simulink model "HIL"  (R2019a)
settings: configuration reference "Configuration" (kept outside this file)
undefined symbols (not defined in the file): Ts
libraries: aerolibutil x2, vrlib x1
settings Model: Creator=zouji  LastModifiedBy=Bingo
settings ConfigSetRef: SourceName=Configuration  SourceLocation=Base Workspace

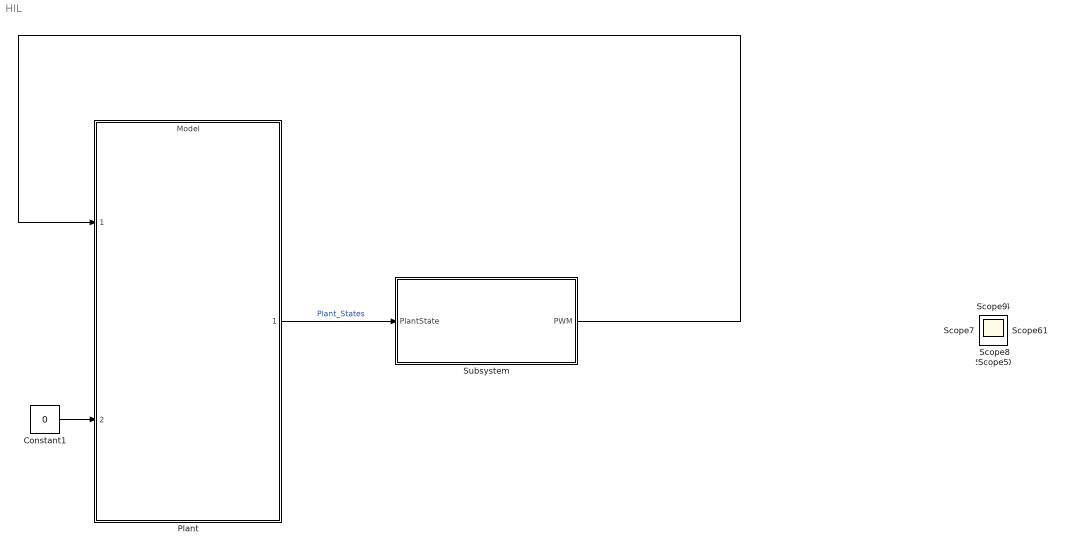
== system HIL ==
  Constant1 : Constant  Value=0  OutDataTypeStr=Inherit: Inherit via back propagation
  Plant : ModelReference  ModelNameDialog=Model.slx  SimulationMode=Normal  ModelReferenceVersion=1.125
  Subsystem : Subsystem
  Scope{,1..11} (12 alike) : Scope
  wires:
  Constant1/1 -> Plant/2
  Subsystem/1(PWM) -> Plant/1
  Plant/1 -> Subsystem/1(PlantState)  "Plant_States"

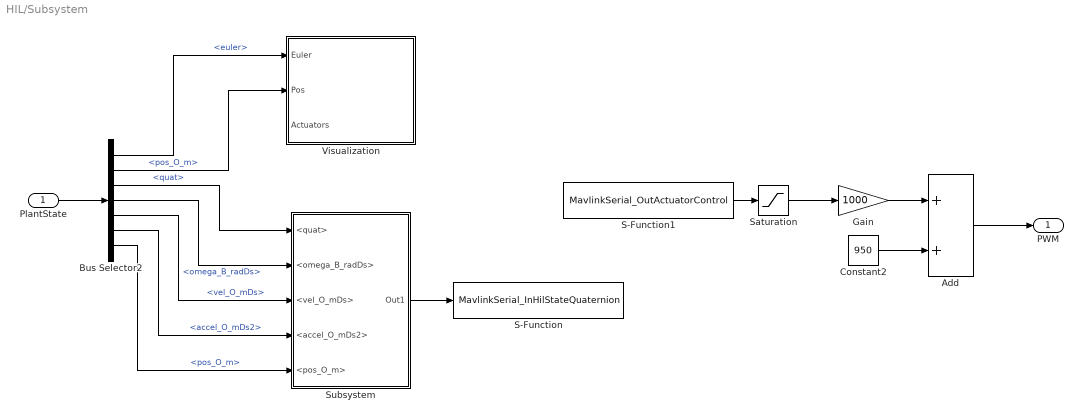
== system HIL/Subsystem ==
  PlantState : Inport
  Add : Sum
  Bus Selector2 : BusSelector  OutputSignals=euler,pos_O_m,quat,omega_B_radDs,vel_O_mDs,accel_O_mDs2,pos_O_m
  Constant2 : Constant  Value=950  OutDataTypeStr=uint16
  Gain : Gain  Gain=1000  OutDataTypeStr=uint16
  S-Function : S-Function  FunctionName=MavlinkSerial_InHilStateQuaternion  SFunctionDeploymentMode=off  EnableBusSupport=off
  S-Function1 : S-Function  FunctionName=MavlinkSerial_OutActuatorControl  SFunctionDeploymentMode=off  EnableBusSupport=off
  Saturation : Saturate  UpperLimit=1  LowerLimit=0
  Subsystem : Subsystem
  Visualization : Subsystem
  PWM : Outport
  wires:
  Add/1 -> PWM/1
  Saturation/1 -> Gain/1
  Constant2/1 -> Add/2
  Gain/1 -> Add/1
  PlantState/1 -> Bus Selector2/1
  S-Function1/1 -> Saturation/1
  Bus Selector2/1 -> Visualization/1(Euler)  "<euler>"
  Bus Selector2/2 -> Visualization/2(Pos)  "<pos_O_m>"
  Bus Selector2/3 -> Subsystem/1(<quat>)  "<quat>"
  Bus Selector2/4 -> Subsystem/2(<omega_B_radDs>)  "<omega_B_radDs>"
  Bus Selector2/5 -> Subsystem/3(<vel_O_mDs>)  "<vel_O_mDs>"
  Bus Selector2/6 -> Subsystem/4(<accel_O_mDs2>)  "<accel_O_mDs2>"
  Bus Selector2/7 -> Subsystem/5(<pos_O_m>)  "<pos_O_m>"
  Subsystem/1(Out1) -> S-Function/1

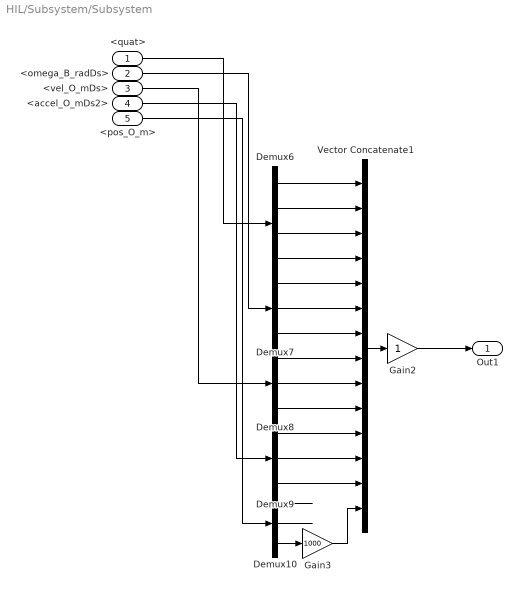
== system HIL/Subsystem/Subsystem ==
  <quat> : Inport
  <omega_B_radDs> : Inport  Port=2
  <vel_O_mDs> : Inport  Port=3
  <accel_O_mDs2> : Inport  Port=4
  <pos_O_m> : Inport  Port=5
  Demux{7..10} (4 alike) : Demux  Outputs=3
  Demux6 : Demux
  Gain2 : Gain  OutDataTypeStr=double
  Gain3 : Gain  Gain=1000
  Vector Concatenate1 : Concatenate  NumInputs=14
  Out1 : Outport
  wires:
  Demux9/2 -> Vector Concatenate1/12
  Gain3/1 -> Vector Concatenate1/14
  Demux6/4 -> Vector Concatenate1/4
  Demux9/1 -> Vector Concatenate1/11
  Gain2/1 -> Out1/1
  Demux8/1 -> Vector Concatenate1/8
  Demux10/3 -> Gain3/1
  Demux9/3 -> Vector Concatenate1/13
  Demux6/1 -> Vector Concatenate1/1
  Demux8/3 -> Vector Concatenate1/10
  Demux7/3 -> Vector Concatenate1/7
  Demux7/1 -> Vector Concatenate1/5
  Vector Concatenate1/1 -> Gain2/1
  Demux7/2 -> Vector Concatenate1/6
  Demux6/3 -> Vector Concatenate1/3
  Demux8/2 -> Vector Concatenate1/9
  Demux10/1 -> ?
  Demux6/2 -> Vector Concatenate1/2
  Demux10/2 -> ?
  <pos_O_m>/1 -> Demux10/1
  <quat>/1 -> Demux6/1
  <vel_O_mDs>/1 -> Demux8/1
  <omega_B_radDs>/1 -> Demux7/1
  <accel_O_mDs2>/1 -> Demux9/1

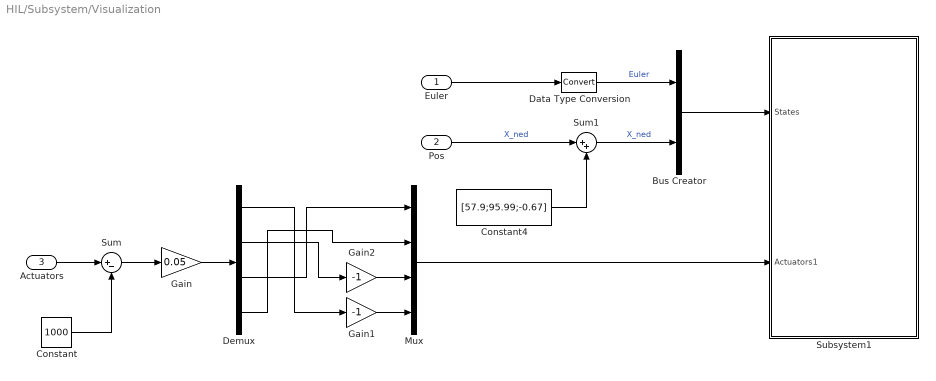
== system HIL/Subsystem/Visualization ==
  Euler : Inport
  Pos : Inport  Port=2
  Actuators : Inport  Port=3
  Bus Creator : BusCreator  Inputs=2
  Constant : Constant  Value=1000  OutDataTypeStr=uint16
  Constant4 : Constant  Value=[57.9;95.99;-0.67]  OutDataTypeStr=Inherit: Inherit via back propagation
  Data Type Conversion : DataTypeConversion
  Demux : Demux
  Gain : Gain  Gain=0.05  OutDataTypeStr=Inherit: Same as input
  Gain1 : Gain  Gain=-1  OutDataTypeStr=Inherit: Same as input
  Gain2 : Gain  Gain=-1  OutDataTypeStr=Inherit: Same as input
  Mux : Mux
  Subsystem1 : Subsystem
  Sum : Sum  Inputs=|+-  OutDataTypeStr=single
  Sum1 : Sum  Inputs=|++
  wires:
  Bus Creator/1 -> Subsystem1/1(States)
  Euler/1 -> Data Type Conversion/1
  Sum1/1 -> Bus Creator/2  "X_ned"
  Actuators/1 -> Sum/1
  Constant/1 -> Sum/2
  Sum/1 -> Gain/1
  Gain/1 -> Demux/1
  Demux/1 -> Gain1/1
  Gain1/1 -> Mux/4
  Demux/2 -> Gain2/1
  Demux/3 -> Mux/1
  Demux/4 -> Mux/2
  Gain2/1 -> Mux/3
  Mux/1 -> Subsystem1/2(Actuators1)
  Constant4/1 -> Sum1/2
  Pos/1 -> Sum1/1  "X_ned"
  Data Type Conversion/1 -> Bus Creator/1  "Euler"

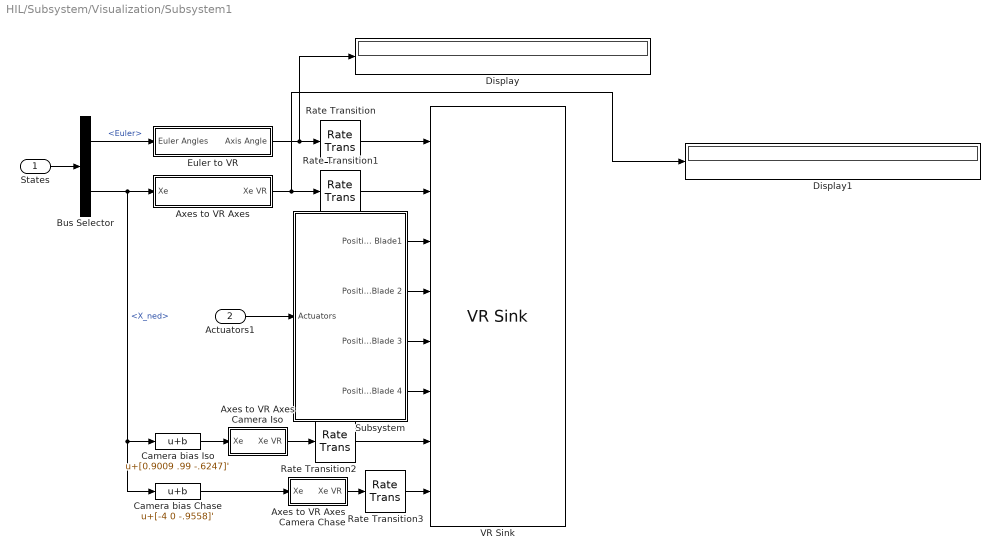
== system HIL/Subsystem/Visualization/Subsystem1 ==
  States : Inport
  Actuators1 : Inport  Port=2
  Axes to VR Axes : Subsystem
  Axes to VR Axes Camera Chase : Subsystem
  Axes to VR Axes Camera Iso : Subsystem
  Bus Selector : BusSelector  OutputSignals=Euler,X_ned
  Camera bias Chase : Bias  Bias=[-4 0 -.9558]'
  Camera bias Iso : Bias  Bias=[0.9009 .99 -.6247]'
  Display : Display
  Display1 : Display
  Euler to VR : Subsystem
  Rate Transition{,1..3} (4 alike) : RateTransition
  Subsystem : Subsystem
  VR Sink : vrlib/VR Sink  InstantiateOnLoad=on  SampleTime=12*Ts  ViewEnable=on  RemoteChange=off  RemoteView=off  FieldsWritten=QuadBody.rotation.4.1.1.double#QuadBody.translation.3.1.1.double#Blade1.rotation.4.1.1.double#Blade3.rotation.4.1.1.double#Blade2.rotation.4.1.1.double#Blade4.rotation.4.1.1.double#IsoNoRotation.position.3.1.1.double#OnQuadNoRotation.position.3.1.1.double  WorldFileName=asbQuadcopterWorld.wrl  AutoView=on  VideoDimensions=[]  AllowVariableSize=off  FigureProperties="{'Position', 'Name', 'Viewpoint', 'CameraBound', 'CameraDirection', 'CameraPosition', 'CameraUpVector', 'ZoomFactor', 'Antialiasing', 'Headlight', 'Lighting', 'NavPanel', 'Sound', 'StatusBar', 'Stereo3D', 'Stereo3DCameraOffset', 'Stereo3DHIT', 'ToolBar', 'Textures', 'Transparency', 'Triad', 'Wireframe', 'NavZones', 'NavMode', 'NavSpeed', 'CaptureFileFormat', 'CaptureFileName', 'Record2DCompressMethod', 'Record2DCompressQuality', 'Record2D', 'Record2DFileName', 'Record2DFPS'; [-1.9190000000000000e+03   1.7500000000000000e+02   1.9200000000000000e+03   9.2200000000000000e+02], '', 'Chase - No Rotation', 'on', [0.0000000000000000e+00   0.0000000000000000e+00  -1.0000000000000000e+00], [0.0000000000000000e+00   0.0000000000000000e+00   0.0000000000000000e+00], [0.0000000000000000e+00   1.0000000000000000e+00   0.0000000000000000e+00], [1.0000000000000000e+00], 'on', 'on', 'on', 'halfbar', 'on', 'on', 'off', [1.0000000149011612e-01], [0.0000000000000000e+00], 'on', 'on', 'on', 'none', 'off', 'off', 'fly', 'normal', 'tif', '%f_anim_%n.tif', 'auto', [7.5000000000000000e+01], 'off', '%f_anim_%n.avi', 'auto'}"
      settings: SourceProductBaseCode=VR
  wires:
  Rate Transition/1 -> VR Sink/1
  Subsystem/3(Position Blade 3) -> VR Sink/5
  States/1 -> Bus Selector/1
  Subsystem/4(Position Blade 4) -> VR Sink/6
  Bus Selector/1 -> Euler to VR/1(Euler Angles)  "<Euler>"
  Camera bias Iso/1 -> Axes to VR Axes Camera Iso/1(Xe)
  Axes to VR Axes/1(Xe VR) -> Display1/1, Rate Transition1/1
  Rate Transition1/1 -> VR Sink/2
  Axes to VR Axes Camera Iso/1(Xe VR) -> Rate Transition2/1
  Bus Selector/2 -> Camera bias Chase/1, Camera bias Iso/1, Axes to VR Axes/1(Xe)  "<X_ned>"
  Axes to VR Axes Camera Chase/1(Xe VR) -> Rate Transition3/1
  Subsystem/2(Position Blade 2) -> VR Sink/4
  Actuators1/1 -> Subsystem/1(Actuators)
  Subsystem/1(Position Blade1) -> VR Sink/3
  Euler to VR/1(Axis Angle) -> Display/1, Rate Transition/1
  Rate Transition3/1 -> VR Sink/8
  Rate Transition2/1 -> VR Sink/7
  Camera bias Chase/1 -> Axes to VR Axes Camera Chase/1(Xe)

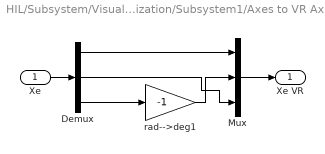
== system HIL/Subsystem/Visualization/Subsystem1/Axes to VR Axes ==
  Xe : Inport
  Demux : Demux  Outputs=3
  Mux : Mux  Inputs=3
  rad-->deg1 : Gain  Gain=-1  SaturateOnIntegerOverflow=on  OutDataTypeStr=Inherit: Same as input  ParamDataTypeStr=Inherit: Same as input
  Xe VR : Outport
  wires:
  Xe/1 -> Demux/1
  Demux/1 -> Mux/1
  Demux/3 -> rad-->deg1/1
  Mux/1 -> Xe VR/1
  rad-->deg1/1 -> Mux/2
  Demux/2 -> Mux/3

== system HIL/Subsystem/Visualization/Subsystem1/Axes to VR Axes Camera Chase ==
  Xe : Inport
  Demux : Demux  Outputs=3
  Mux : Mux  Inputs=3
  rad-->deg1 : Gain  Gain=-1  SaturateOnIntegerOverflow=on  OutDataTypeStr=Inherit: Same as input  ParamDataTypeStr=Inherit: Same as input
  Xe VR : Outport
  wires:
  Xe/1 -> Demux/1
  Demux/1 -> Mux/1
  Demux/3 -> rad-->deg1/1
  Mux/1 -> Xe VR/1
  rad-->deg1/1 -> Mux/2
  Demux/2 -> Mux/3

== system HIL/Subsystem/Visualization/Subsystem1/Axes to VR Axes Camera Iso ==
  Xe : Inport
  Demux : Demux  Outputs=3
  Mux : Mux  Inputs=3
  rad-->deg1 : Gain  Gain=-1  SaturateOnIntegerOverflow=on  OutDataTypeStr=Inherit: Same as input  ParamDataTypeStr=Inherit: Same as input
  Xe VR : Outport
  wires:
  Demux/2 -> Mux/3
  rad-->deg1/1 -> Mux/2
  Mux/1 -> Xe VR/1
  Demux/3 -> rad-->deg1/1
  Demux/1 -> Mux/1
  Xe/1 -> Demux/1

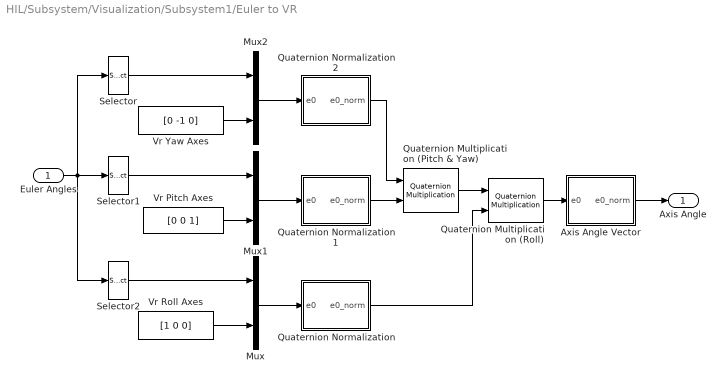
== system HIL/Subsystem/Visualization/Subsystem1/Euler to VR ==
  Euler Angles : Inport
  Axis Angle Vector : Subsystem
  Mux : Mux  Inputs=2
  Mux1 : Mux  Inputs=2
  Mux2 : Mux  Inputs=2
  Quaternion Multiplication (Pitch & Yaw) : aerolibutil/Quaternion Multiplication
  Quaternion Multiplication (Roll) : aerolibutil/Quaternion Multiplication
  Quaternion Normalization : Subsystem
  Quaternion Normalization1 : Subsystem
  Quaternion Normalization2 : Subsystem
  Selector : Selector  InputPortWidth=3  IndexOptions=Index vector (dialog)  Indices=[3]  OutputSizes=1
  Selector1 : Selector  InputPortWidth=3  IndexOptions=Index vector (dialog)  Indices=[2]  OutputSizes=1
  Selector2 : Selector  InputPortWidth=3  IndexOptions=Index vector (dialog)  Indices=[1]  OutputSizes=1
  Vr Pitch Axes : Constant  Value=[0 0 1]
  Vr Roll Axes : Constant  Value=[1 0 0]
  Vr Yaw Axes : Constant  Value=[0 -1 0]
  Axis Angle : Outport
  wires:
  Quaternion Multiplication (Roll)/1 -> Axis Angle Vector/1(e0)
  Axis Angle Vector/1(e0_norm) -> Axis Angle/1
  Quaternion Normalization/1(e0_norm) -> Quaternion Multiplication (Roll)/2
  Quaternion Normalization2/1(e0_norm) -> Quaternion Multiplication (Pitch & Yaw)/1
  Quaternion Normalization1/1(e0_norm) -> Quaternion Multiplication (Pitch & Yaw)/2
  Mux2/1 -> Quaternion Normalization2/1(e0)
  Mux1/1 -> Quaternion Normalization1/1(e0)
  Mux/1 -> Quaternion Normalization/1(e0)
  Selector/1 -> Mux2/1
  Vr Yaw Axes/1 -> Mux2/2
  Selector1/1 -> Mux1/1
  Vr Pitch Axes/1 -> Mux1/2
  Selector2/1 -> Mux/1
  Vr Roll Axes/1 -> Mux/2
  Euler Angles/1 -> Selector2/1, Selector1/1, Selector/1
  Quaternion Multiplication (Pitch & Yaw)/1 -> Quaternion Multiplication (Roll)/1

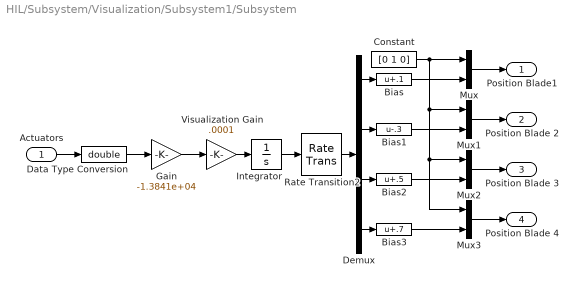
== system HIL/Subsystem/Visualization/Subsystem1/Subsystem ==
  Actuators : Inport
  Bias : Bias  Bias=.1
  Bias1 : Bias  Bias=-.3
  Bias2 : Bias  Bias=.5
  Bias3 : Bias  Bias=.7
  Constant : Constant  Value=[0 1 0]
  Data Type Conversion : DataTypeConversion  OutDataTypeStr=double
  Demux : Demux
  Gain : Gain  Gain=-1.3841e+04
  Integrator : Integrator  InitialCondition="[.1  .2 -.3 -.4]"  WrapState=on  WrappedStateUpperValue=2*pi  WrappedStateLowerValue=-2*pi
  Mux{,1..3} (4 alike) : Mux  Inputs=2
  Rate Transition2 : RateTransition
  Visualization Gain : Gain  Gain=.0001
  Position Blade1 : Outport
  Position Blade 2 : Outport  Port=2
  Position Blade 3 : Outport  Port=3
  Position Blade 4 : Outport  Port=4
  wires:
  Bias3/1 -> Mux3/2
  Mux3/1 -> Position Blade 4/1
  Bias1/1 -> Mux1/2
  Bias2/1 -> Mux2/2
  Demux/2 -> Bias1/1
  Visualization Gain/1 -> Integrator/1
  Constant/1 -> Mux3/1, Mux2/1, Mux1/1, Mux/1
  Mux1/1 -> Position Blade 2/1
  Mux2/1 -> Position Blade 3/1
  Data Type Conversion/1 -> Gain/1
  Integrator/1 -> Rate Transition2/1
  Mux/1 -> Position Blade1/1
  Gain/1 -> Visualization Gain/1
  Demux/3 -> Bias2/1
  Bias/1 -> Mux/2
  Actuators/1 -> Data Type Conversion/1
  Demux/4 -> Bias3/1
  Rate Transition2/1 -> Demux/1
  Demux/1 -> Bias/1

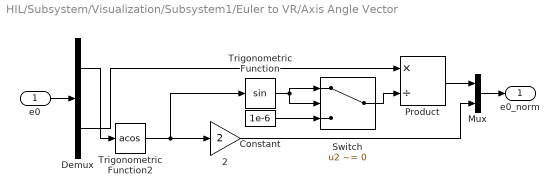
== system HIL/Subsystem/Visualization/Subsystem1/Euler to VR/Axis Angle Vector ==
  e0 : Inport
  2 : Gain  Gain=2  SaturateOnIntegerOverflow=on  OutDataTypeStr=Inherit: Same as input  ParamDataTypeStr=Inherit: Same as input
  Constant : Constant  Value=1e-6
  Demux : Demux  Outputs=[1 3 ]
  Mux : Mux  Inputs=2
  Product : Product  Inputs=*/  SaturateOnIntegerOverflow=on  InputSameDT=on  OutDataTypeStr=Inherit: Same as first input
  Switch : Switch  Criteria=u2 ~= 0
  Trigonometric Function : Trigonometry
  Trigonometric Function2 : Trigonometry  Operator=acos
  e0_norm : Outport
  wires:
  Demux/1 -> Trigonometric Function2/1
  Demux/2 -> Product/1
  Mux/1 -> e0_norm/1
  Product/1 -> Mux/1
  2/1 -> Mux/2
  Trigonometric Function/1 -> Switch/1, Switch/2
  Trigonometric Function2/1 -> Trigonometric Function/1, 2/1
  e0/1 -> Demux/1
  Constant/1 -> Switch/3
  Switch/1 -> Product/2

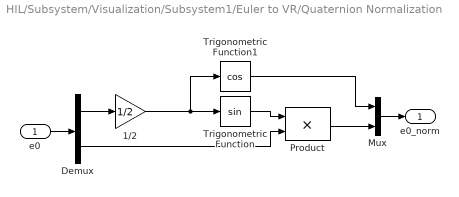
== system HIL/Subsystem/Visualization/Subsystem1/Euler to VR/Quaternion Normalization ==
  e0 : Inport
  1/2 : Gain  Gain=1/2  SaturateOnIntegerOverflow=on  OutDataTypeStr=Inherit: Same as input  ParamDataTypeStr=Inherit: Same as input
  Demux : Demux  Outputs=[1 3]
  Mux : Mux  Inputs=2
  Product : Product  SaturateOnIntegerOverflow=on  InputSameDT=on  OutDataTypeStr=Inherit: Same as first input
  Trigonometric Function : Trigonometry
  Trigonometric Function1 : Trigonometry  Operator=cos
  e0_norm : Outport
  wires:
  Trigonometric Function1/1 -> Mux/1
  Demux/2 -> Product/2
  Demux/1 -> 1/2/1
  Mux/1 -> e0_norm/1
  Product/1 -> Mux/2
  Trigonometric Function/1 -> Product/1
  1/2/1 -> Trigonometric Function1/1, Trigonometric Function/1
  e0/1 -> Demux/1

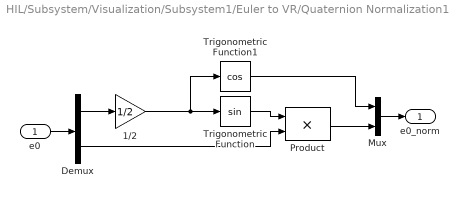
== system HIL/Subsystem/Visualization/Subsystem1/Euler to VR/Quaternion Normalization1 ==
  e0 : Inport
  1/2 : Gain  Gain=1/2  SaturateOnIntegerOverflow=on  OutDataTypeStr=Inherit: Same as input  ParamDataTypeStr=Inherit: Same as input
  Demux : Demux  Outputs=[1 3]
  Mux : Mux  Inputs=2
  Product : Product  SaturateOnIntegerOverflow=on  InputSameDT=on  OutDataTypeStr=Inherit: Same as first input
  Trigonometric Function : Trigonometry
  Trigonometric Function1 : Trigonometry  Operator=cos
  e0_norm : Outport
  wires:
  e0/1 -> Demux/1
  1/2/1 -> Trigonometric Function/1, Trigonometric Function1/1
  Trigonometric Function/1 -> Product/1
  Product/1 -> Mux/2
  Mux/1 -> e0_norm/1
  Demux/1 -> 1/2/1
  Demux/2 -> Product/2
  Trigonometric Function1/1 -> Mux/1

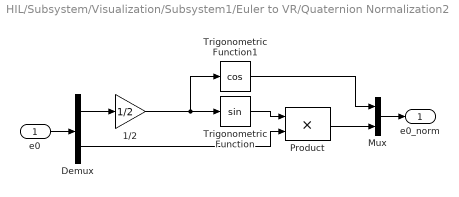
== system HIL/Subsystem/Visualization/Subsystem1/Euler to VR/Quaternion Normalization2 ==
  e0 : Inport
  1/2 : Gain  Gain=1/2  SaturateOnIntegerOverflow=on  OutDataTypeStr=Inherit: Same as input  ParamDataTypeStr=Inherit: Same as input
  Demux : Demux  Outputs=[1 3]
  Mux : Mux  Inputs=2
  Product : Product  SaturateOnIntegerOverflow=on  InputSameDT=on  OutDataTypeStr=Inherit: Same as first input
  Trigonometric Function : Trigonometry
  Trigonometric Function1 : Trigonometry  Operator=cos
  e0_norm : Outport
  wires:
  Trigonometric Function1/1 -> Mux/1
  Demux/2 -> Product/2
  Demux/1 -> 1/2/1
  Mux/1 -> e0_norm/1
  Product/1 -> Mux/2
  Trigonometric Function/1 -> Product/1
  1/2/1 -> Trigonometric Function1/1, Trigonometric Function/1
  e0/1 -> Demux/1
